simulink model "q3"  (R2020b)
settings: Solver=FixedStepAuto  StartTime=0.0  StopTime=10.0  RelTol=1e-3
undefined symbols (not defined in the file): c1, c2
settings Model: Creator=AVM  LastModifiedBy=AVM

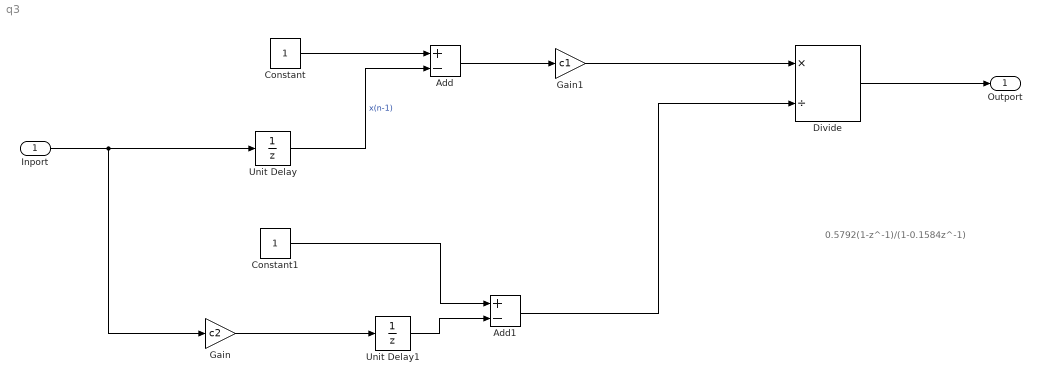
== system q3 ==
  note: 0.5792(1-z^-1)/(1-0.1584z^-1)
  Inport : Inport
  Add : Sum  Inputs=+-
  Add1 : Sum  Inputs=+-
  Constant : Constant
  Constant1 : Constant
  Divide : Product  Inputs=*/
  Gain : Gain  Gain=c2
  Gain1 : Gain  Gain=c1
  Unit Delay : UnitDelay  SampleTime=-1  HasFrameUpgradeWarning=on
  Unit Delay1 : UnitDelay  SampleTime=-1  HasFrameUpgradeWarning=on
  Outport : Outport
  wires:
  Divide/1 -> Outport/1
  Add1/1 -> Divide/2
  Gain1/1 -> Divide/1
  Add/1 -> Gain1/1
  Constant/1 -> Add/1
  Unit Delay1/1 -> Add1/2
  Gain/1 -> Unit Delay1/1
  Inport/1 -> Gain/1, Unit Delay/1
  Unit Delay/1 -> Add/2  "x(n-1)"
  Constant1/1 -> Add1/1
